simulink model "velocity_form_mpc2024A"  (R2024a)
settings: Solver=VariableStepAuto  StartTime=0.0  StopTime=1  RelTol=1e-3
values from neighbouring files (symbols this model uses):
  N = 5    [project_script.m]    (also in scriptpoint7.m)
  NK = 0    [scriptpoint7.m]
  Qd = 1*eye(2)    [project_script.m]    (also in scriptpoint7.m = 1000*eye(2))
  Rd = 1*eye(2)    [project_script.m]    (also in scriptpoint7.m)
  RK = 1*eye(2)    [scriptpoint7.m]
  Ts = 1/8000    (= 0.000125)    [project_script.m]    (also in scriptpoint7.m)
  u_bar_d = Bd\ (eye(size(Ad))-Ad)*xref    [project_script.m]    (also in scriptpoint7.m)
  u_sat_max = [u1_max; u2_max]    [project_script.m]    (also in scriptpoint7.m)
  u_sat_min = [u1_min; u2_min]    [project_script.m]    (also in scriptpoint7.m)
  x0 = [x0_1;x0_2]    [project_script.m]    (also in scriptpoint7.m)
  x_sat_max = [x1_max; x2_max]    [project_script.m]    (also in scriptpoint7.m)
  x_sat_min = [x1_min; x2_min]    [project_script.m]    (also in scriptpoint7.m)
  xref = [6.9; 8.9]    [project_script.m]    (also in scriptpoint7.m)
undefined symbols (not defined in the file or in its folder): Ad, Ad_real, Bd, Bd_real, Cd, Cd_real, Dd, Dd_real, Discrete, myvelocitympc, Sd, Time
libraries: ctrlSharedLib x1
settings Model: Creator=andre  LastModifiedBy=Utente

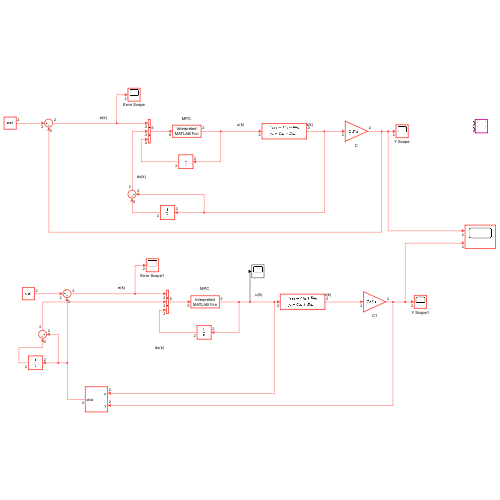
[thumbnail: Simulink's stored preview of the top-level diagram]
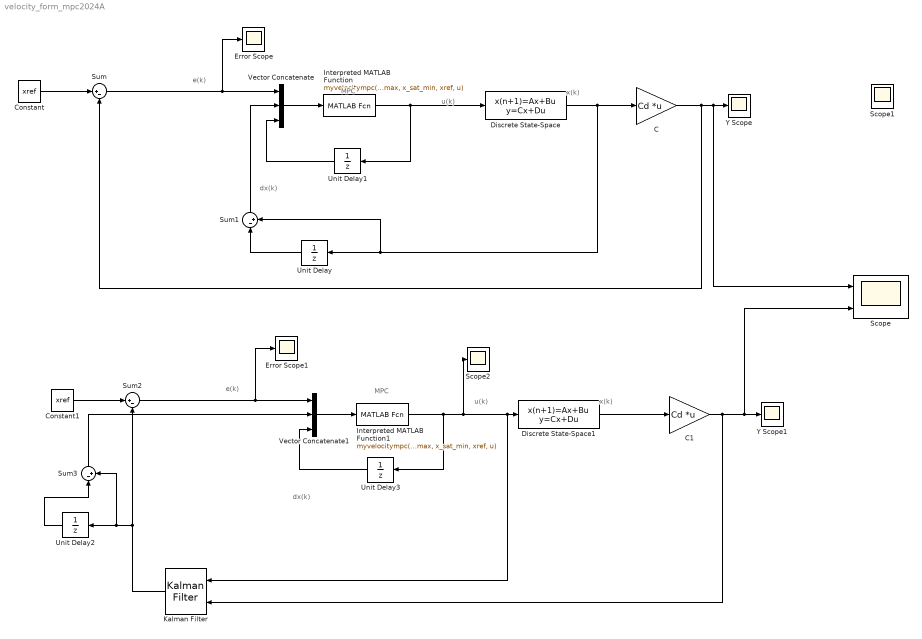
== system velocity_form_mpc2024A ==
  note: u(k)
  note: x(k)
  note: dx(k)
  note: e(k)
  note: MPC
  note: x(k)
  note: dx(k)
  note: u(k)
  note: MPC
  note: e(k)
  C : Gain  Gain=Cd  Multiplication=Matrix(K*u)
  C1 : Gain  Gain=Cd  Multiplication=Matrix(K*u)
  Constant : Constant  Value=xref  SampleTime=Ts
  Constant1 : Constant  Value=xref  SampleTime=Ts
  Discrete State-Space : DiscreteStateSpace  A=Ad  B=Bd  C=Cd  D=Dd  InitialCondition=x0  SampleTime=Ts
  Discrete State-Space1 : DiscreteStateSpace  A=Ad_real  B=Bd_real  C=Cd_real  D=Dd_real  InitialCondition=x0  SampleTime=Ts
  Error Scope : Scope
  Error Scope1 : Scope
  Interpreted MATLAB Function : MATLABFcn  MATLABFcn=myvelocitympc(Ad,Bd,Cd,Qd,Rd,Sd,N,u_sat_min,u_sat_max,u_bar_d, x_sat_max, x_sat_min, xref, u)  OutputDimensions=2
  Interpreted MATLAB Function1 : MATLABFcn  MATLABFcn=myvelocitympc(Ad,Bd,Cd,Qd,Rd,Sd,N,u_sat_min,u_sat_max,u_bar_d, x_sat_max, x_sat_min, xref, u)  OutputDimensions=2
  Kalman Filter : ctrlSharedLib/Kalman Filter  TimeDomain=Discrete-Time  UseCurrentEstimator=on  ModelSource=Individual A, B, C, D matrices  ModelSourceVariable=ss(0.95,1,1,0,1)  A=Ad  B=Bd  C=Cd  D=Dd  NumberOfStates=1  NumberOfInputs=1  NumberOfOutputs=1  InitialEstimateSource=Dialog  X0=0  P0=10  UseK=off  UseGH=off  NumberOfProcessNoiseInputs=1  G=1  TimeInvariantG=on  H=0  TimeInvariantH=on  Q=QK  TimeInvariantQ=on  R=RK  TimeInvariantR=on  N=NK  TimeInvariantN=on  AddInputPort=on  AddEnablePort=off  OutputEstimatedY=off  OutputP=off  Ts=Ts
  Scope : Scope  NumInputPorts=2
  Scope1 : Scope  NumInputPorts=2
  Scope2 : Scope
  Sum : Sum  Inputs=|+-
  Sum1 : Sum  Inputs=|-+
  Sum2 : Sum  Inputs=|+-
  Sum3 : Sum  Inputs=|-+
  Unit Delay{,1..3} (4 alike) : UnitDelay  SampleTime=Ts  HasFrameUpgradeWarning=on
  Vector Concatenate : Concatenate  NumInputs=3
  Vector Concatenate1 : Concatenate  NumInputs=3
  Y Scope : Scope
  Y Scope1 : Scope
  wires:
  C/1 -> Sum/2, Scope/1, Y Scope/1
  Constant/1 -> Sum/1
  Discrete State-Space/1 -> Sum1/2, Unit Delay/1, C/1
  Unit Delay/1 -> Sum1/1
  Interpreted MATLAB Function/1 -> Discrete State-Space/1, Unit Delay1/1
  Sum1/1 -> Vector Concatenate/2
  Sum/1 -> Error Scope/1, Vector Concatenate/1
  Vector Concatenate/1 -> Interpreted MATLAB Function/1
  Unit Delay1/1 -> Vector Concatenate/3
  Discrete State-Space1/1 -> C1/1
  Unit Delay3/1 -> Vector Concatenate1/3
  Unit Delay2/1 -> Sum3/1
  C1/1 -> Kalman Filter/2, Scope/2, Y Scope1/1
  Vector Concatenate1/1 -> Interpreted MATLAB Function1/1
  Sum2/1 -> Error Scope1/1, Vector Concatenate1/1
  Constant1/1 -> Sum2/1
  Sum3/1 -> Vector Concatenate1/2
  Kalman Filter/1 -> Sum3/2, Unit Delay2/1, Sum2/2
  Interpreted MATLAB Function1/1 -> Scope2/1, Kalman Filter/1, Discrete State-Space1/1, Unit Delay3/1
